simulink model "HybridVehicle_PIL"  (R2020b)
settings: Solver=ode23tb  StartTime=0.0  StopTime=1800  RelTol=1e-3
model workspace (MAT data in the model file):
  DownShiftSpeeds = [11.05  11.05  11.05  11.05  11.05  11.05  11.05  11.05  11.05  11.05  11.05  11.05  19.55  25.5  31.45  35.7  35.7; 18.7  18.7  18.7  18.7  19.125  20.48636  21.33636  23.375  27.28636  30.26136  33.827365  38.76136  46.072635  56.1  64.6  73.1  73.1; 28.9  28.9  28.9  28.9  28.9  30.51364  34.51136  41.56364  47.68636  53.377365  58.477365  65.622635  73.525  81.26136  88.48636  115.6  115.6; 38.675  38.675  38.675  38.675  39.43864  42.41364  47.68636  56.43864  65.11136  72.927365  80.497635  90.01364  100.81136  110.672635  122.4  153  153; 51.425  51.425  51.425  51.425  51.76364  55.077365  62.38864  72.422635  83.3  102  136  425  425  425  425  425  425]
  I = 0.25
  Kbr = 1000000
  MGUMaxPower = 50000
  P = 15
  PedalPositions = [0 6.2485 12.4969 18.7454 24.9939 31.2424 37.4908 43.7393 49.9878 56.2363 62.4847 68.7332 74.9817 81.2302 87.4786 93.7271 99.9756]
  SOCmax = 99
  TrqICMax = 175
  TrqMGUMax = 150
  TrqMax = 325
  UpShiftSpeeds = [12.75  12.75  12.75  12.75  12.75  12.75  15.552365  17.08636  18.7  20.227365  23.46136  27.625  31.702365  36.63636  42.5  42.5  42.5; 20.997635  20.997635  20.997635  20.997635  21.927365  24.902365  28.727365  31.78864  35.275  39.697635  46.41136  51.85  59.672635  67.48864  78.2  78.2  78.2; 31.45  31.45  31.45  31.45  34.172635  41.052365  47.175  52.952365  59.5  68  76.5  85  93.5  106.25  119.85  119.85  119.85; 42.16136  42.16136  42.16136  43.947635  47.002365  54.31364  63.325  71.227365  79.222635  88.06136  98.852365  109.052365  118.402365  128.86136  157.25  157.25  157.25; 55.58864  55.58864  55.58864  58.052365  61.53864  72.077365  85.51136  96.81364  255  255  255  255  255  255  255  255  255]
  axle_b = 10
  axle_k = 5000
  bevAxle_wc = 400
  bevNp = 2
  bevNs = 30
  brkTrqMGU = 150
  brkTrqMax = 700
  convAxle_wc = 500
  diffRatio = 3.4
  diffRatio1 = 3.4
  driveshaft_b = 10
  driveshaft_k = 2500
  driveshaft_wc = 500
  engineSpeedPoints_rpm = [750 1053.57142857 1357.14285714 1660.71428571 1964.28571429 2267.85714286 2571.42857143 2875 3178.57142857 3482.14285714 3785.71428571 4089.28571429 4392.85714286 4696.42857143 5000]
  engineTorqueMap_Nm = [-13.6738264269 15.0034460821 26.4289521305 37.8539339756 49.2854604964 60.7146317399 72.0173711595 77.7345012802 77.7345012802 77.7345012802 77.7345012802 77.7345012802 ... (240 elements, 16x15)]
  engineTorquePoints_Nm = [0 15 26.4285714286 37.8571428571 49.2857142857 60.7142857143 72.1428571429 83.5714285714 95 106.428571429 117.857142857 129.285714286 140.714285714 152.142857143 163.571428571 175]
  fuelCapacity = 35
  motorMaxTorqueNm = [500 500 500 500 500 500 416.666666667 357.142857143 312.5 277.777777778 250 227.272727273 208.333333333 192.307692308 178.571428571 166.666666667]
  motorSpeedRadPs = [0 40 80 120 160 200 240 280 320 360 400 440 480 520 560 600]
  tau_IC = 2
  tau_Regen = 1
  vehicleMass = 1500
  wheelRadius = 0.35
libraries: eeGeneralControl x2, autolibshared x2, pil_lib x1
settings Model: SILPILModeSetting=veronly  ExtModeTrigDuration=2  Creator=ivane  LastModifiedBy=galli
settings OptimizationCC: PassReuseOutputArgsAs=Individual arguments  ZeroExternalMemoryAtStartup=off  ZeroInternalMemoryAtStartup=off  MaxStackSize=64  OptimizationLevel=level1  OptimizationCustomize=off  EfficientTunableParamExpr=on
settings DebuggingCC: ParameterTunabilityLossMsg=error
settings HardwareCC: ProdBitPerInt=16  ProdBitPerPointer=16  ProdBitPerSizeT=16  ProdBitPerPtrDiffT=16  ProdLargestAtomicFloat=None  ProdWordSize=8  ProdHWDeviceType=Atmel->AVR
settings SFSimCC: MATLABDynamicMemAlloc=off
settings RTWCC: Description=Embedded Coder  SystemTargetFile=ert.tlc  HardwareBoard=Arduino Uno  TemplateMakefile=ert_default_tmf  Toolchain=Arduino AVR  BuildConfiguration=Faster Runs  CreateSILPILBlock=PIL
settings CodeAppCC: ForceParamTrailComments=on  IgnoreCustomStorageClasses=off  OperatorAnnotations=on  SimulinkDataObjDesc=on  SFDataObjDesc=on  InsertBlockDesc=on
settings ERTTargetCC: SupportContinuousTime=on  SupportVariableSizeSignals=on  ExtModeStaticAllocSize=250

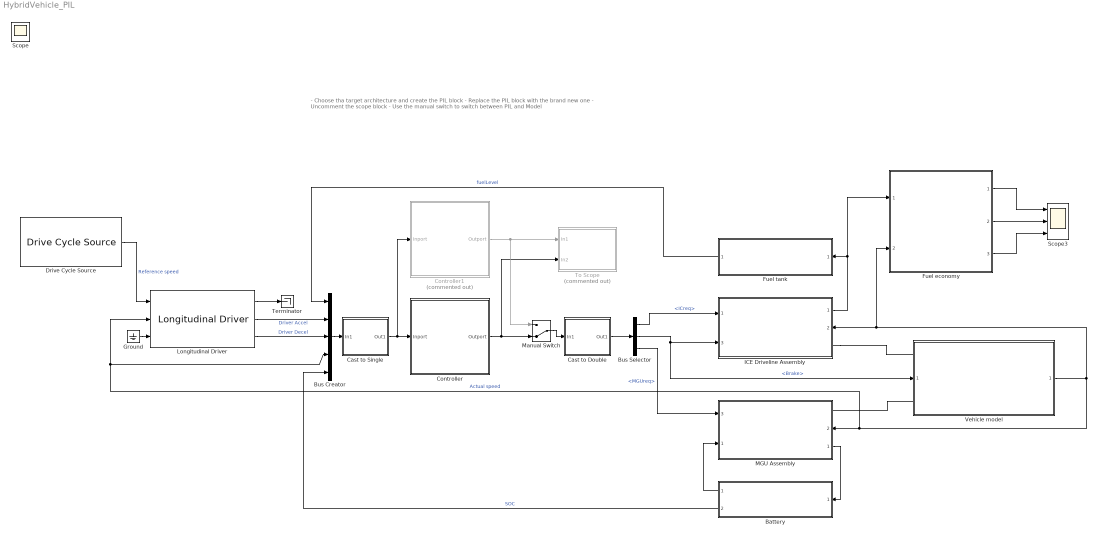
== system HybridVehicle_PIL ==
  note: - Choose tha target architecture and create the PIL block
      | - Replace the PIL block with the brand new one
      | - Uncomment the scope block
      | - Use the manual switch to switch between PIL and Model
  Battery : Subsystem  ReferencedSubsystem=Battery
      settings: PortSchema="{\"entries\":[{\"content\":{\"sides\":[{\"content\":{\"connectorIds\":[\"Out1\",\"Out2\"]},\"type\":\"ConnectorPlacement.EquallySpacedRectSide\",\"uuid\":\"62c661fb-2963-4729-8409-c11ca18452bb\"},{\"content\":{\"connectorIds\":[\"In1\"],\"side\":\"RIGHT\"},\"type\":\"ConnectorPlacement.EquallySpacedRectSide\",\"uuid\":\"8d8a0df4-31a2-4844-b6e4-fdfd8750374f\"},{\"content\":{\"connectorIds\":[],\"side\":\"TOP\"},\"type\":\"ConnectorPlacement.EquallySpacedRectSide\",\"uuid\":\"345d14b7-5d59-4ed6-ba31-c78cc2155fc5\"},{\"content\":{\"connectorIds\":[],\"side\":\"HIDDEN\"},\"type\":\"ConnectorPlacement.EquallySpacedRectSide\",\"uuid\":\"be681e4d-0788-4d60-9432-78c6b7c184d6\"}]},\"type\":\"ConnectorPlacement.EquallySpacedConnector\",\"uuid\":\"76d22945-58a4-4f01-9ad4-fc5d192e1319\"}],\"packageUris\":[\"http://schema.mathworks.com/mf0/Connector/R2020b\"],\"version\":\"1.0\"}"
  Bus Creator : BusCreator  Inputs=5
  Bus Selector : BusSelector  OutputSignals=ICreq,Brake,MGUreq
  Cast to Double : Subsystem
  Cast to Single : Subsystem
  Controller : Subsystem  TreatAsAtomicUnit=on
  Controller1 : Subsystem  Commented=on  DialogController=pil_create_dialog  LoadFcn=|
      | try
      |    if ~strcmp(rtw.pil.getPILVersion, '9.9 (R2020b)_14')
      |       set_param(gcb, 'DialogController', '');
      |       set_param(gcb, 'DialogControllerArgs', '');
      |    end
      | catch e
      |       set_param(gcb, 'DialogController', '');
      |       set_param(gcb, 'DialogControllerArgs', '');
      | end
      mask help: PIL:pil:XILBlockMaskDesc
      mask Display: disp('PIL');
  Drive Cycle Source : autolibshared/Drive Cycle Source  cycleVar=Workspace variable  wsVar=WLTP_class_3  fileVar=cycleFTP75.mat  tfinal="1800  seconds"  cycleRepeat=off  outAccPort=off  outGearPort=off  gearList=No gear data  t_wot1=5  xdot_woto=0  xdot_wot1=30  t_wot2=20  xdot_wot2=0  t_wotend=30  srcUnit=km/h  outUnit=km/h  srcAccUnit=m/s/s  outAccUnit=m/s^2  dt=0  aMode=1  faultOption=off  velBnd=2  velBndUnit=mph  inUnit=m/s  timeBnd=1  failOption=off  stopSim=off  maxFaultCnt=10  maxFaultTime=2  maxTotFaultTime=15  traceOption=off  dtTrace=1  traceWindow=10  lastDCname=Custom Data Set 1  lastOutUnit=mph  lastDT=0  lastTB=1  lastSB=2  forceCalcBound=off
      settings: SourceProductBaseCode=PW,MT,UV,VE,VP
  Fuel economy : Subsystem  ReferencedSubsystem=Fuel_economy
  Fuel tank : Subsystem  ReferencedSubsystem=fuelTank
  Ground : Ground
  ICE Driveline Assembly : Subsystem  ReferencedSubsystem=IC_Driveline
      settings: PortSchema="{\"entries\":[{\"content\":{\"sides\":[{\"content\":{\"connectorIds\":[\"In1\",\"In3\"]},\"type\":\"ConnectorPlacement.EquallySpacedRectSide\",\"uuid\":\"d2a2af2f-0810-46c5-a89d-1fb3bffb58b0\"},{\"content\":{\"connectorIds\":[\"Out1\",\"In2\",\"RConn1\"],\"side\":\"RIGHT\"},\"type\":\"ConnectorPlacement.EquallySpacedRectSide\",\"uuid\":\"5d91c2bd-bc93-425c-9733-5ba49e3ee9da\"},{\"content\":{\"connectorIds\":[],\"side\":\"TOP\"},\"type\":\"ConnectorPlacement.EquallySpacedRectSide\",\"uuid\":\"30272aa7-5431-486b-ba2d-786d8a62fe2e\"},{\"content\":{\"connectorIds\":[],\"side\":\"HIDDEN\"},\"type\":\"ConnectorPlacement.EquallySpacedRectSide\",\"uuid\":\"f07e1d6c-3558-4c7b-844c-ecaea33e0b73\"}]},\"type\":\"ConnectorPlacement.EquallySpacedConnector\",\"uuid\":\"e11bd347-ea62-4e54-9941-5a9032f6c7d6\"}],\"packageUris\":[\"http://schema.mathworks.com/mf0/Connector/R2020b\"],\"version\":\"1.0\"}"
  Longitudinal Driver : autolibshared/Longitudinal Driver  extAccelOvr=off  extDecelOvr=off  extAccelHld=off  extDecelHld=off  extAccelZero=off  extDecelZero=off  cntrlType=PI  shftType=None  velUnits=km/h  gearOut=off  Kp=15  Ki=0.5  Kff=0  Kg=0  VehVelVec=[0 100]  KffVec=[.1 .1]  KpVec=[10 10]  KiVec=[5 5]  KgVec=[0 0]  m=1500  Kpt=3000  tau=.1  L=2  aR=200  bR=2.5  cR=.5  g=9.81  vnom=100  Kaw=0  tauerr=.0  tauPt=2  GearInit=0  tShift=.1  pdlVec=[0.1 0.4 0.5 0.9]  upShftTbl=[-1 12.9375 26.4375 39.9375 51.18749999999999 62.4375 72.84375 83.25;-1 16.3125 29.8125 43.3125 54.5624 65.8125 76.78125 87.75;-1 19.6875 33.1875 46.68749999999999 57.9375 69.1875 80.71875 92.25;-1 33 52.5 77.25 100.5 138.75 161.875 185]  dwnShftTbl=[1 9.5625 23.0625 36.5625 47.8125 59.0625 68.90625 78.75;1 12.9375 26.4375 39.9375 51.18749999999999 62.4375 72.84375 83.25;1 16.3125 29.8125 43.3125 54.562499 65.8125 76.78125 87.75;1 19.6875 33.1875 46.68749999999999 57.9375 69.1875 80.71875 92.25]  tClutch=.5  tRev=.5  tPark=120  aMode=1  UpGearVec="[0  1  2  3  4  5  6  7]"  DownGearVec="[1  2  3  4  5  6  7  8]"
      settings: SourceProductBaseCode=PW,MT,UV,VE,VP
  MGU Assembly : Subsystem  ReferencedSubsystem=MGU
      settings: PortSchema="{\"entries\":[{\"content\":{\"sides\":[{\"content\":{\"connectorIds\":[\"In3\",\"In1\"]},\"type\":\"ConnectorPlacement.EquallySpacedRectSide\",\"uuid\":\"d2a2af2f-0810-46c5-a89d-1fb3bffb58b0\"},{\"content\":{\"connectorIds\":[\"RConn1\",\"In2\",\"Out1\"],\"side\":\"RIGHT\"},\"type\":\"ConnectorPlacement.EquallySpacedRectSide\",\"uuid\":\"5d91c2bd-bc93-425c-9733-5ba49e3ee9da\"},{\"content\":{\"connectorIds\":[],\"side\":\"TOP\"},\"type\":\"ConnectorPlacement.EquallySpacedRectSide\",\"uuid\":\"30272aa7-5431-486b-ba2d-786d8a62fe2e\"},{\"content\":{\"connectorIds\":[],\"side\":\"HIDDEN\"},\"type\":\"ConnectorPlacement.EquallySpacedRectSide\",\"uuid\":\"f07e1d6c-3558-4c7b-844c-ecaea33e0b73\"}]},\"type\":\"ConnectorPlacement.EquallySpacedConnector\",\"uuid\":\"e11bd347-ea62-4e54-9941-5a9032f6c7d6\"}],\"packageUris\":[\"http://schema.mathworks.com/mf0/Connector/R2020b\"],\"version\":\"1.0\"}"
  Manual Switch : ManualSwitch  CurrentSetting=0
  Scope3 : Scope  NumInputPorts=3
  Terminator : Terminator
  To Scope : Subsystem  Commented=on
  Vehicle model : Subsystem  ReferencedSubsystem=vehicleModel
      settings: PortSchema="{\"entries\":[{\"content\":{\"sides\":[{\"content\":{\"connectorIds\":[\"LConn1\",\"In1\",\"LConn2\"]},\"type\":\"ConnectorPlacement.EquallySpacedRectSide\",\"uuid\":\"297baffa-e0bc-4afe-8d3b-fef71b7412b4\"},{\"content\":{\"connectorIds\":[\"Out1\"],\"side\":\"RIGHT\"},\"type\":\"ConnectorPlacement.EquallySpacedRectSide\",\"uuid\":\"8a12a35b-b522-4ba0-9ba0-852b497f573e\"},{\"content\":{\"connectorIds\":[],\"side\":\"TOP\"},\"type\":\"ConnectorPlacement.EquallySpacedRectSide\",\"uuid\":\"b4b51f6d-39af-472b-beff-f9410fe777e8\"},{\"content\":{\"connectorIds\":[],\"side\":\"HIDDEN\"},\"type\":\"ConnectorPlacement.EquallySpacedRectSide\",\"uuid\":\"ccc4846e-18b0-46b1-8b77-dbf40ce11e43\"}]},\"type\":\"ConnectorPlacement.EquallySpacedConnector\",\"uuid\":\"224bfd92-7422-4b82-8ee3-7d4031b335e8\"}],\"packageUris\":[\"http://schema.mathworks.com/mf0/Connector/R2020b\"],\"version\":\"1.0\"}"
  Scope : Scope
  wires:
  Longitudinal Driver/2 -> Bus Creator/2  "Driver Accel"
  Longitudinal Driver/3 -> Bus Creator/3  "Driver Decel"
  Bus Selector/1 -> ICE Driveline Assembly/1  "<ICreq>"
  Fuel tank/1 -> Bus Creator/1  "fuelLevel"
  ICE Driveline Assembly/1 -> Fuel economy/1, Fuel tank/1
  MGU Assembly/1 -> Battery/1
  Battery/1 -> MGU Assembly/1
  Battery/2 -> Bus Creator/5  "SOC"
  Vehicle model/1 -> MGU Assembly/2, Longitudinal Driver/2, Bus Creator/4, Fuel economy/2, ICE Driveline Assembly/2  "Actual speed"
  Drive Cycle Source/1 -> Longitudinal Driver/1  "Reference speed"
  Ground/1 -> Longitudinal Driver/3
  Longitudinal Driver/1 -> Terminator/1
  Fuel economy/3 -> Scope3/3
  Fuel economy/1 -> Scope3/1
  Fuel economy/2 -> Scope3/2
  Bus Selector/2 -> Vehicle model/1, ICE Driveline Assembly/3  "<Brake>"
  Bus Selector/3 -> MGU Assembly/3  "<MGUreq>"
  Bus Creator/1 -> Cast to Single/1(In1)
  Cast to Single/1(Out1) -> Controller1/1(Inport), Controller/1(Inport)
  Cast to Double/1(Out1) -> Bus Selector/1
  Controller/1(Outport) -> To Scope/2(In2), Manual Switch/2
  Manual Switch/1 -> Cast to Double/1(In1)
  Controller1/1(Outport) -> Manual Switch/1, To Scope/1(In1)
  connections:
  ICE Driveline Assembly/RConn1 -- Vehicle model/LConn1
  Vehicle model/LConn2 -- MGU Assembly/RConn1

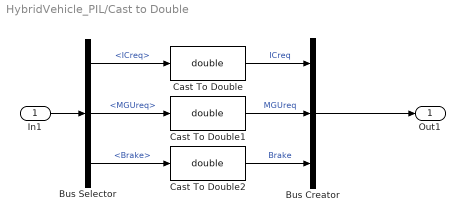
== system HybridVehicle_PIL/Cast to Double ==
  In1 : Inport
  Bus Creator : BusCreator  Inputs=3
  Bus Selector : BusSelector  OutputSignals=ICreq,MGUreq,Brake
  Cast To Double : DataTypeConversion  OutDataTypeStr=double
  Cast To Double1 : DataTypeConversion  OutDataTypeStr=double
  Cast To Double2 : DataTypeConversion  OutDataTypeStr=double
  Out1 : Outport
  wires:
  In1/1 -> Bus Selector/1
  Bus Selector/1 -> Cast To Double/1  "<ICreq>"
  Bus Selector/2 -> Cast To Double1/1  "<MGUreq>"
  Bus Selector/3 -> Cast To Double2/1  "<Brake>"
  Cast To Double/1 -> Bus Creator/1  "ICreq"
  Cast To Double1/1 -> Bus Creator/2  "MGUreq"
  Cast To Double2/1 -> Bus Creator/3  "Brake"
  Bus Creator/1 -> Out1/1

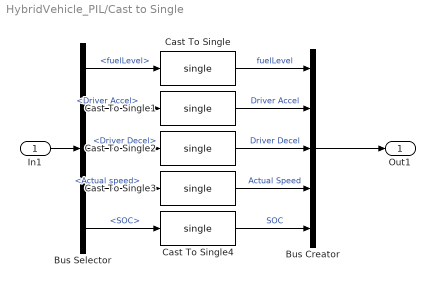
== system HybridVehicle_PIL/Cast to Single ==
  In1 : Inport
  Bus Creator : BusCreator  Inputs=5
  Bus Selector : BusSelector  OutputSignals=fuelLevel,Driver Accel,Driver Decel,Actual speed,SOC
  Cast To Single{,1..4} (5 alike) : DataTypeConversion  OutDataTypeStr=single
  Out1 : Outport
  wires:
  In1/1 -> Bus Selector/1
  Bus Selector/1 -> Cast To Single/1  "<fuelLevel>"
  Bus Selector/2 -> Cast To Single1/1  "<Driver Accel>"
  Bus Selector/3 -> Cast To Single2/1  "<Driver Decel>"
  Bus Selector/4 -> Cast To Single3/1  "<Actual speed>"
  Bus Selector/5 -> Cast To Single4/1  "<SOC>"
  Cast To Single/1 -> Bus Creator/1  "fuelLevel"
  Cast To Single1/1 -> Bus Creator/2  "Driver Accel"
  Cast To Single2/1 -> Bus Creator/3  "Driver Decel"
  Cast To Single3/1 -> Bus Creator/4  "Actual Speed"
  Cast To Single4/1 -> Bus Creator/5  "SOC"
  Bus Creator/1 -> Out1/1

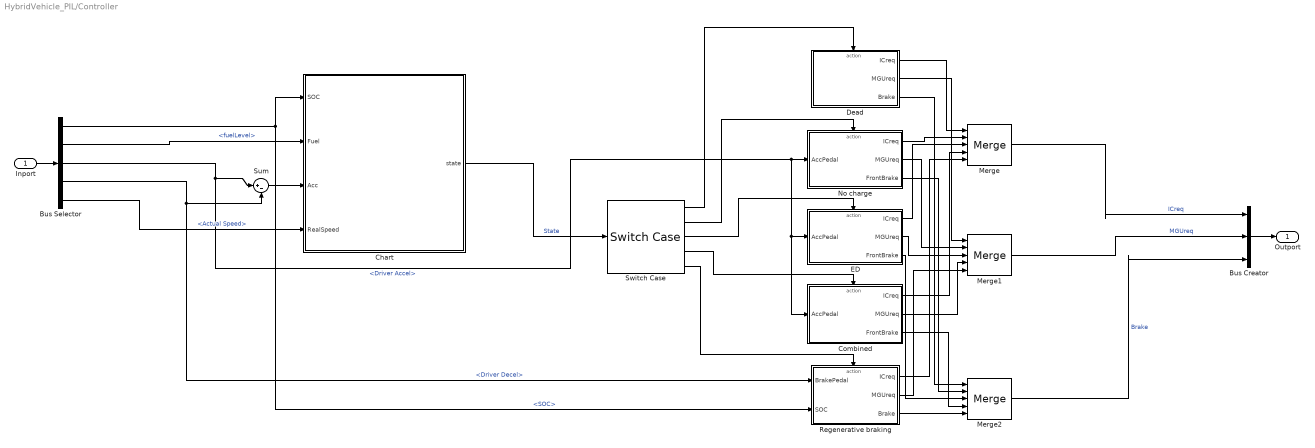
== system HybridVehicle_PIL/Controller ==
  Inport : Inport
  Bus Creator : BusCreator  Inputs=3
  Bus Selector : BusSelector  OutputSignals=SOC,fuelLevel,Driver Accel,Driver Decel,Actual Speed
  Chart : Stateflow chart  TreatAsAtomicUnit=on
  Combined : Subsystem  TreatAsAtomicUnit=on
  Dead : Subsystem  TreatAsAtomicUnit=on
  ED : Subsystem  TreatAsAtomicUnit=on
  Merge : Merge  Inputs=5
  Merge1 : Merge  Inputs=5
  Merge2 : Merge  Inputs=5
  No charge : Subsystem  TreatAsAtomicUnit=on
  Regenerative braking : Subsystem  TreatAsAtomicUnit=on
  Sum : Sum  Inputs=|+-
  Switch Case : SwitchCase  CaseConditions={0,1,2,3,4}  ShowDefaultCase=off
  Outport : Outport
  wires:
  Merge/1 -> Bus Creator/1  "ICreq"
  Merge1/1 -> Bus Creator/2  "MGUreq"
  Merge2/1 -> Bus Creator/3  "Brake"
  Chart/1(state) -> Switch Case/1  "State"
  Sum/1 -> Chart/3(Acc)
  Dead/3(Brake) -> Merge2/1
  ED/1(ICreq) -> Merge/3
  ED/3(FrontBrake) -> Merge2/3
  Dead/1(ICreq) -> Merge/1
  Regenerative braking/1(ICreq) -> Merge/5
  No charge/1(ICreq) -> Merge/2
  Bus Selector/1 -> Chart/1(SOC), Regenerative braking/2(SOC)  "<SOC>"
  Regenerative braking/2(MGUreq) -> Merge1/5
  ED/2(MGUreq) -> Merge1/3
  Combined/2(MGUreq) -> Merge1/4
  No charge/3(FrontBrake) -> Merge2/2
  Switch Case/1 -> Dead/Action
  Switch Case/3 -> ED/Action
  Switch Case/5 -> Regenerative braking/Action
  Switch Case/2 -> No charge/Action
  Combined/1(ICreq) -> Merge/4
  No charge/2(MGUreq) -> Merge1/2
  Dead/2(MGUreq) -> Merge1/1
  Combined/3(FrontBrake) -> Merge2/4
  Regenerative braking/3(Brake) -> Merge2/5
  Switch Case/4 -> Combined/Action
  Inport/1 -> Bus Selector/1
  Bus Selector/2 -> Chart/2(Fuel)  "<fuelLevel>"
  Bus Selector/3 -> Sum/1, Combined/1(AccPedal), ED/1(AccPedal), No charge/1(AccPedal)  "<Driver Accel>"
  Bus Selector/4 -> Sum/2, Regenerative braking/1(BrakePedal)  "<Driver Decel>"
  Bus Selector/5 -> Chart/4(RealSpeed)  "<Actual Speed>"
  Bus Creator/1 -> Outport/1

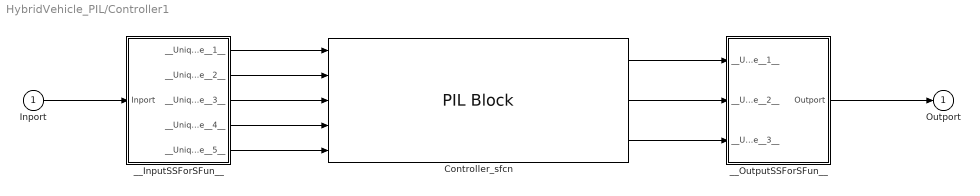
== system HybridVehicle_PIL/Controller1 ==
  Inport : Inport
  Controller_sfcn : pil_lib/PIL Block  SimulationMode=PIL  IsTopModelPIL=off  CodeDir=<binary blob, 123 chars, not shown>  AnchorDir=/Users/francescoprignoli/Documents/MATLAB/CoDeAS/hybrid-controller/Hybrid-controller/Simulation/PIL/Code  ConfigName=Arduino Board  XrelIsTopModelCode=on  XrelIsReusable=off  XrelDWorkNames={}  XrelDWorkTypes={}  XrelModelArgVals={}  XrelOrderedParamNames={}
      settings: SourceProductBaseCode=RT
  __InputSSForSFun__ : Subsystem
  __OutputSSForSFun__ : Subsystem
  Outport : Outport
  wires:
  Inport/1 -> __InputSSForSFun__/1(Inport)
  __InputSSForSFun__/1(__UniqueOutportName__1__) -> Controller_sfcn/1
  __InputSSForSFun__/2(__UniqueOutportName__2__) -> Controller_sfcn/2
  __InputSSForSFun__/3(__UniqueOutportName__3__) -> Controller_sfcn/3
  __InputSSForSFun__/4(__UniqueOutportName__4__) -> Controller_sfcn/4
  __InputSSForSFun__/5(__UniqueOutportName__5__) -> Controller_sfcn/5
  Controller_sfcn/1 -> __OutputSSForSFun__/1(__UniqueInportName__1__)
  Controller_sfcn/2 -> __OutputSSForSFun__/2(__UniqueInportName__2__)
  Controller_sfcn/3 -> __OutputSSForSFun__/3(__UniqueInportName__3__)
  __OutputSSForSFun__/1(Outport) -> Outport/1

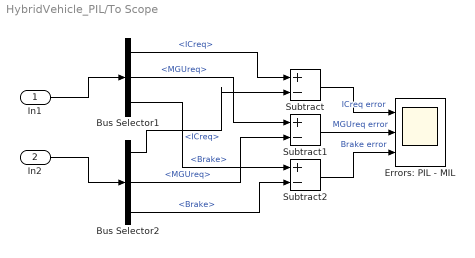
== system HybridVehicle_PIL/To Scope ==
  In1 : Inport
  In2 : Inport  Port=2
  Bus Selector1 : BusSelector  OutputSignals=ICreq,MGUreq,Brake
  Bus Selector2 : BusSelector  OutputSignals=ICreq,MGUreq,Brake
  Errors: PIL - MIL : Scope  NumInputPorts=3
  Subtract : Sum  Inputs=+-
  Subtract1 : Sum  Inputs=+-
  Subtract2 : Sum  Inputs=+-
  wires:
  Bus Selector1/2 -> Subtract1/1  "<MGUreq>"
  In1/1 -> Bus Selector1/1
  Bus Selector2/2 -> Subtract1/2  "<MGUreq>"
  Bus Selector2/1 -> Subtract/2  "<ICreq>"
  In2/1 -> Bus Selector2/1
  Bus Selector1/1 -> Subtract/1  "<ICreq>"
  Bus Selector1/3 -> Subtract2/1  "<Brake>"
  Bus Selector2/3 -> Subtract2/2  "<Brake>"
  Subtract1/1 -> Errors: PIL - MIL/2  "MGUreq error"
  Subtract/1 -> Errors: PIL - MIL/1  "ICreq error"
  Subtract2/1 -> Errors: PIL - MIL/3  "Brake error"

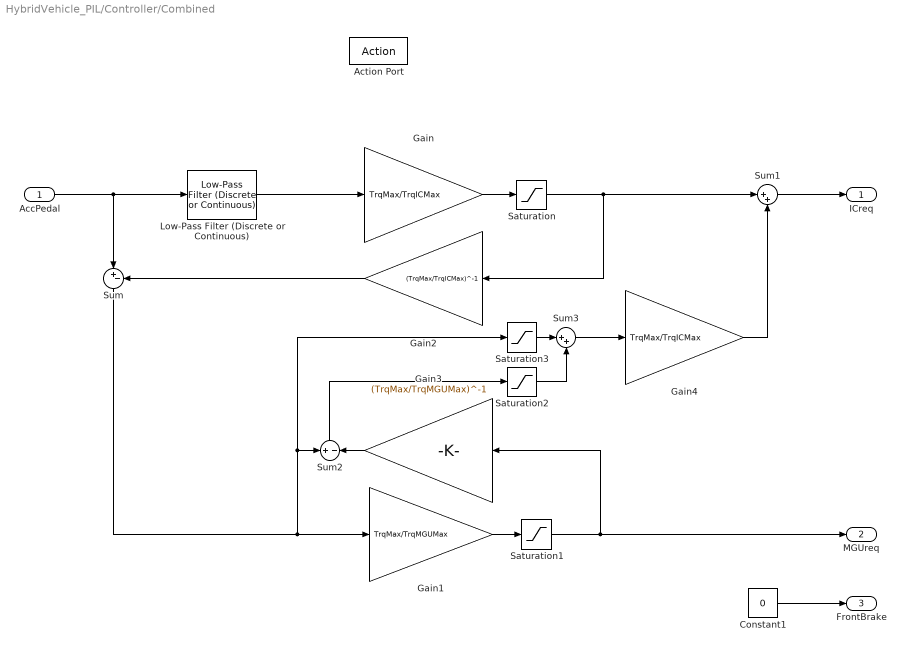
== system HybridVehicle_PIL/Controller/Combined ==
  AccPedal : Inport
  Action Port : ActionPort  InitializeStates=reset  ActionPortLabel=case [ 3 ]:
  Constant1 : Constant  Value=0  OutDataTypeStr=single
  Gain : Gain  Gain=TrqMax/TrqICMax  OutDataTypeStr=single
  Gain1 : Gain  Gain=TrqMax/TrqMGUMax  OutDataTypeStr=single
  Gain2 : Gain  Gain=(TrqMax/TrqICMax)^-1  OutDataTypeStr=single
  Gain3 : Gain  Gain=(TrqMax/TrqMGUMax)^-1  OutDataTypeStr=single
  Gain4 : Gain  Gain=TrqMax/TrqICMax  OutDataTypeStr=single
  Low-Pass Filter (Discrete or Continuous) : eeGeneralControl/Low-Pass Filter (Discrete or Continuous)  K=1  T=tau_IC  B=inf  A=-inf  init_option=Specify as parameter  x0=0  Ts=-1
  Saturation : Saturate  UpperLimit=1  LowerLimit=0
  Saturation1 : Saturate  UpperLimit=1  LowerLimit=0
  Saturation2 : Saturate  UpperLimit=1  LowerLimit=0
  Saturation3 : Saturate  UpperLimit=0  LowerLimit=-1
  Sum : Sum  Inputs=|+-
  Sum1 : Sum  Inputs=|++
  Sum2 : Sum  Inputs=+|-
  Sum3 : Sum  Inputs=|++
  ICreq : Outport
  MGUreq : Outport  Port=2
  FrontBrake : Outport  Port=3
  wires:
  Gain2/1 -> Sum/2
  Gain3/1 -> Sum2/2
  Low-Pass Filter (Discrete or Continuous)/1 -> Gain/1
  Saturation1/1 -> MGUreq/1, Gain3/1
  Gain1/1 -> Saturation1/1
  Gain/1 -> Saturation/1
  Sum/1 -> Gain1/1, Saturation3/1, Sum2/1
  Sum1/1 -> ICreq/1
  Sum2/1 -> Saturation2/1
  Saturation3/1 -> Sum3/1
  Sum3/1 -> Gain4/1
  Saturation2/1 -> Sum3/2
  Constant1/1 -> FrontBrake/1
  Gain4/1 -> Sum1/2
  AccPedal/1 -> Sum/1, Low-Pass Filter (Discrete or Continuous)/1
  Saturation/1 -> Sum1/1, Gain2/1

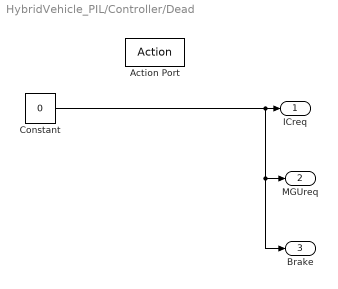
== system HybridVehicle_PIL/Controller/Dead ==
  Action Port : ActionPort  InitializeStates=reset  ActionPortLabel=case [ 0 ]:
  Constant : Constant  Value=0  OutDataTypeStr=single
  ICreq : Outport
  MGUreq : Outport  Port=2
  Brake : Outport  Port=3
  wires:
  Constant/1 -> ICreq/1, Brake/1, MGUreq/1

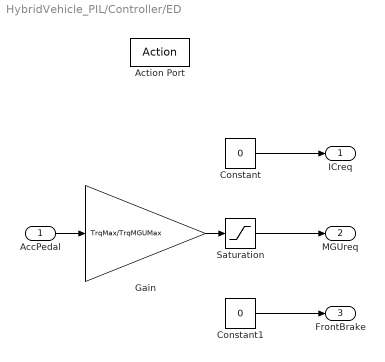
== system HybridVehicle_PIL/Controller/ED ==
  AccPedal : Inport
  Action Port : ActionPort  InitializeStates=reset  ActionPortLabel=case [ 2 ]:
  Constant : Constant  Value=0  OutDataTypeStr=single
  Constant1 : Constant  Value=0  OutDataTypeStr=single
  Gain : Gain  Gain=TrqMax/TrqMGUMax
  Saturation : Saturate  UpperLimit=1  LowerLimit=0
  ICreq : Outport
  MGUreq : Outport  Port=2
  FrontBrake : Outport  Port=3
  wires:
  Saturation/1 -> MGUreq/1
  Gain/1 -> Saturation/1
  AccPedal/1 -> Gain/1
  Constant/1 -> ICreq/1
  Constant1/1 -> FrontBrake/1

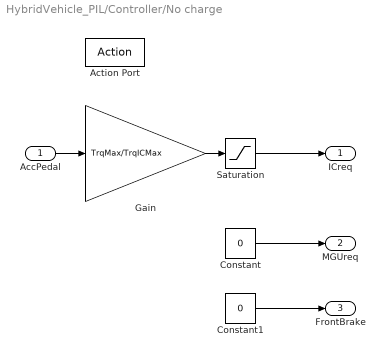
== system HybridVehicle_PIL/Controller/No charge ==
  AccPedal : Inport
  Action Port : ActionPort  InitializeStates=reset  ActionPortLabel=case [ 1 ]:
  Constant : Constant  Value=0  OutDataTypeStr=single
  Constant1 : Constant  Value=0  OutDataTypeStr=single
  Gain : Gain  Gain=TrqMax/TrqICMax
  Saturation : Saturate  UpperLimit=1  LowerLimit=0
  ICreq : Outport
  MGUreq : Outport  Port=2
  FrontBrake : Outport  Port=3
  wires:
  Constant/1 -> MGUreq/1
  Saturation/1 -> ICreq/1
  AccPedal/1 -> Gain/1
  Gain/1 -> Saturation/1
  Constant1/1 -> FrontBrake/1

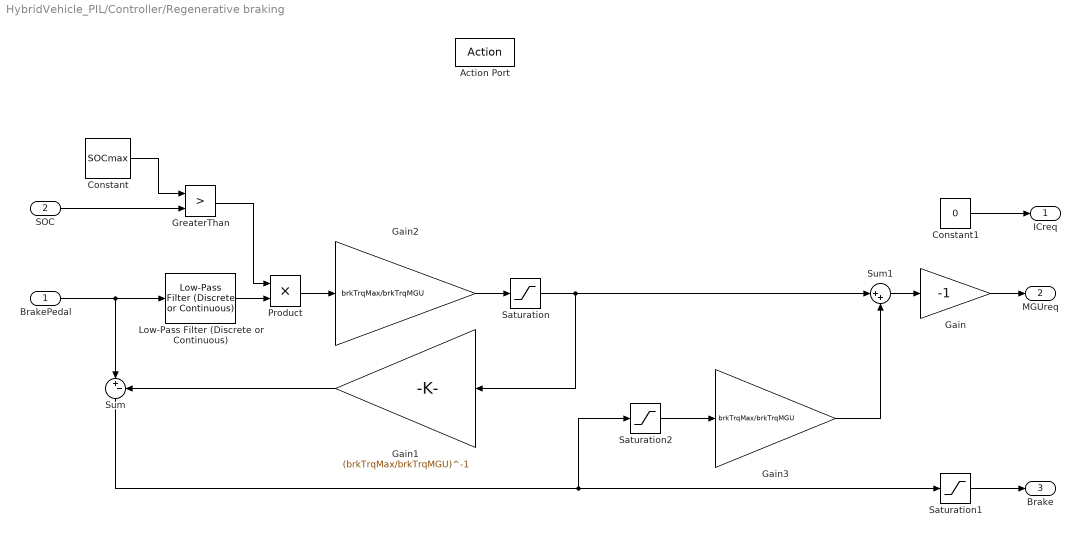
== system HybridVehicle_PIL/Controller/Regenerative braking ==
  BrakePedal : Inport
  SOC : Inport  Port=2
  Action Port : ActionPort  InitializeStates=reset  ActionPortLabel=case [ 4 ]:
  Constant : Constant  Value=SOCmax
  Constant1 : Constant  Value=0  OutDataTypeStr=single
  Gain : Gain  Description=added a gain about -0.65 to introduce the concept of efficency in the regenerative braking  Gain=-1  OutDataTypeStr=single
  Gain1 : Gain  Gain=(brkTrqMax/brkTrqMGU)^-1  OutDataTypeStr=single
  Gain2 : Gain  Gain=brkTrqMax/brkTrqMGU  OutDataTypeStr=single
  Gain3 : Gain  Gain=brkTrqMax/brkTrqMGU  OutDataTypeStr=single
  GreaterThan : RelationalOperator  Operator=>  OutDataTypeStr=fixdt(1,16)  RndMeth=Simplest
  Low-Pass Filter (Discrete or Continuous) : eeGeneralControl/Low-Pass Filter (Discrete or Continuous)  K=1  T=1  B=inf  A=-inf  init_option=Specify as parameter  x0=0  Ts=-1
  Product : Product
  Saturation : Saturate  UpperLimit=1  LowerLimit=0
  Saturation1 : Saturate  UpperLimit=1  LowerLimit=0
  Saturation2 : Saturate  UpperLimit=0  LowerLimit=-1
  Sum : Sum  Inputs=|+-
  Sum1 : Sum  Inputs=|++
  ICreq : Outport
  MGUreq : Outport  Port=2
  Brake : Outport  Port=3
  wires:
  GreaterThan/1 -> Product/1
  Gain1/1 -> Sum/2
  Product/1 -> Gain2/1
  Low-Pass Filter (Discrete or Continuous)/1 -> Product/2
  Saturation/1 -> Gain1/1, Sum1/1
  Gain2/1 -> Saturation/1
  Sum/1 -> Saturation2/1, Saturation1/1
  BrakePedal/1 -> Low-Pass Filter (Discrete or Continuous)/1, Sum/1
  Saturation1/1 -> Brake/1
  SOC/1 -> GreaterThan/2
  Constant/1 -> GreaterThan/1
  Constant1/1 -> ICreq/1
  Gain/1 -> MGUreq/1
  Saturation2/1 -> Gain3/1
  Gain3/1 -> Sum1/2
  Sum1/1 -> Gain/1

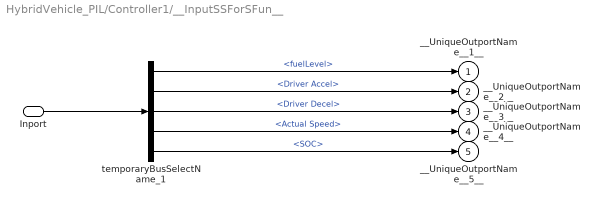
== system HybridVehicle_PIL/Controller1/__InputSSForSFun__ ==
  Inport : Inport
  temporaryBusSelectName_1 : BusSelector  OutputSignals=fuelLevel,Driver Accel,Driver Decel,Actual Speed,SOC
  __UniqueOutportName__1__ : Outport
  __UniqueOutportName__2__ : Outport  Port=2
  __UniqueOutportName__3__ : Outport  Port=3
  __UniqueOutportName__4__ : Outport  Port=4
  __UniqueOutportName__5__ : Outport  Port=5
  wires:
  Inport/1 -> temporaryBusSelectName_1/1
  temporaryBusSelectName_1/1 -> __UniqueOutportName__1__/1  "<fuelLevel>"
  temporaryBusSelectName_1/2 -> __UniqueOutportName__2__/1  "<Driver Accel>"
  temporaryBusSelectName_1/3 -> __UniqueOutportName__3__/1  "<Driver Decel>"
  temporaryBusSelectName_1/4 -> __UniqueOutportName__4__/1  "<Actual Speed>"
  temporaryBusSelectName_1/5 -> __UniqueOutportName__5__/1  "<SOC>"

== system HybridVehicle_PIL/Controller1/__OutputSSForSFun__ ==
  __UniqueInportName__1__ : Inport
  __UniqueInportName__2__ : Inport  Port=2
  __UniqueInportName__3__ : Inport  Port=3
  Mux1 : BusCreator  Inputs=3
  Outport : Outport
  wires:
  __UniqueInportName__1__/1 -> Mux1/1  "ICreq"
  __UniqueInportName__2__/1 -> Mux1/2  "MGUreq"
  __UniqueInportName__3__/1 -> Mux1/3  "Brake"
  Mux1/1 -> Outport/1

== stateflow chart HybridVehicle_PIL/Controller/Chart ==
  settings: updateMethod=DISCRETE  sampleTime=0.01
  state Dead
    %Dead state. It occurs when there is no fuel in the tank and not charge in the battery
    state = 0;
  state NoCharge
    %occurs when the battery SOC is under a treshold. The car switch full ICE
    state=1;
  state ED
    %Electric drive. Occurs when forced by the city zone of under a reference speed
    %imponi v<vedmax se non vi è benzina
    state=2;
  state Combined
    %)(Hybrid drive) over a certain spped both the engine will collaborate to give the required torque
    %IMPONI V<VEDmin se finisce il carburante prima di andare in ED
    state=3;
  state Rigenerative_Braking
    %you will go in that state every time you brake. So the acceleration will be lower than zero.
    %this will so charge the battery til to reach the SOCmax that will limit my case
    state=4;
  Rigenerative_Braking -> Dead [order 2] : [(SOC < SOCmin+SOCth) && (Fuel<fuelMin+fuelHys) ]
  (default) -> Dead
  Dead -> Rigenerative_Braking [order 1] : [Acc<0]
  Dead -> NoCharge [order 4] : [ (Fuel>fuelMin+fuelHys)]
  Dead -> ED [order 3] : [(SOC > SOCmin+SOCth)]
  NoCharge -> Dead [order 2] : [(Fuel<fuelMin+fuelHys) && (SOC <=SOCmin+SOCth)]
  ED -> Dead [order 2] : [(SOC<SOCmin+SOCth) && (Fuel<fuelMin+fuelHys) ]
  Combined -> Dead [order 2] : [(Fuel<fuelMin+fuelHys) && (SOC <=SOCmin+SOCth)]
  Dead -> Combined [order 2] : [(SOC > SOCmin+SOCth) && (Acc>maxAccICE || Acc>maxAccMGU) && (Fuel>fuelMin+fuelHys)]
  ED -> NoCharge [order 3] : [(Fuel>fuelMin+fuelHys) && (SOC <=SOCmin+SOCth)]
  Rigenerative_Braking -> NoCharge [order 4] : [ (Fuel>fuelMin+fuelHys)&& (SOC < SOCmin+SOCth)]
  NoCharge -> ED [order 3] : [((SOC > SOCmin+SOCth) && (RealSpeed < SpeedEDmax)) || ((Fuel<fuelMin+fuelHys) && (SOC >SOCmin+SOCth))]
  NoCharge -> Rigenerative_Braking [order 1] : [Acc<0]
  Combined -> NoCharge [order 4] : [(SOC <= SOCmin + SOCth)&&(Fuel>fuelMin+fuelHys)]
  NoCharge -> Combined [order 4] : [(SOC > SOCmin+SOCth) && (Fuel>fuelMin+fuelHys) &&Acc>maxAccICE]
  ED -> Combined [order 4] : [((RealSpeed>=SpeedEDmax)&& (Fuel>fuelMin+fuelHys))|| ((Fuel>fuelMin+fuelHys)  && Acc>maxAccMGU)]
  Combined -> ED [order 3] : [(RealSpeed<SpeedEDmax)&& (SOC >SOCmin+SOCth)&&Acc<maxAccMGU]
  Rigenerative_Braking -> ED [order 3] : [(SOC > SOCmin+SOCth) && (RealSpeed<SpeedEDmax)]
  ED -> Rigenerative_Braking [order 1] : [Acc<0]
  Combined -> Rigenerative_Braking [order 1] : [Acc < 0]
  Rigenerative_Braking -> Combined [order 5] : [(SOC > SOCmin+SOCth) && (RealSpeed>SpeedEDmax) && (Fuel>fuelMin+fuelHys)]
  Rigenerative_Braking -> Rigenerative_Braking [order 1] : [Acc<0]
  data: SOC input; Fuel input; Acc input; RealSpeed input; state output; SpeedEDmax constant single =45; fuelMin constant single =0.33; SOCth constant single =5; SOCmin constant single =10; fuelHys constant single =0.17; maxAccICE constant single =TrqICMax/TrqMax; maxAccMGU constant single =TrqMGUMax/TrqMax
